simulink model "OML58_Cores"  (R2021b)
settings: Solver=ode4  StartTime=0.0  StopTime=inf  FixedStep=Ts  RelTol=1e-3  EnableMultiTasking=on
PostLoadFcn:
  | Ts = 50e-6;
InitFcn:
  | Ts = 50e-6;
undefined symbols (not defined in the file): I, Left, Right, type, V
libraries: spsSeriesRLCBranchLib x24, spsThreePhaseSeriesRLCLoadLib x12, spsThreePhaseSeriesRLCBranchLib x12, spsThreePhaseBreakerLib x12, artemis x10, spsGroundLib x8, rtlab x6, LafaeLib x6, spsThreePhaseTransformerTwoWindingsLib x5, spsThreePhaseVIMeasurementLib x5, spsPower3phInstantaneousLib x3, spsThreePhaseSourceLib x1
(part 1 of 3)
Description:
  | Model of a simple control system for use iin training.
settings Model: ARTEMISmethode_block_infos=$$__separator__$$OML58_Cores/ARTEMIS Guide$$__separator__$$  Creator=Paul Baracos  LastModifiedBy=lafae
settings SolverCC: AlgebraicLoopSolver=TrustRegion
settings DataIOCC: LimitDataPoints=on  SaveFormat=Array  SignalLoggingSaveFormat=ModelDataLogs  SaveOutput=off  SaveTime=off  ReturnWorkspaceOutputs=off  SignalLoggingName=sigsOut
settings OptimizationCC: BlockReduction=off  BooleanDataType=off  OptimizeBlockIOStorage=off  BufferReuse=off  ExpressionFolding=off  LocalBlockOutputs=off  InitFltsAndDblsToZero=on  LifeSpan=inf
settings DebuggingCC: SaveWithParameterizedLinksMsg=none  UnderspecifiedInitializationDetection=Classic  MergeDetectMultiDrivingBlocksExec=none  SignalResolutionControl=TryResolveAllWithWarning  MultiTaskDSMMsg=warning  MultiTaskCondExecSysMsg=none  FcnCallInpInsideContextMsg=warning  SFUnexpectedBacktrackingDiag=warning  SFNoUnconditionalDefaultTransitionDiag=warning  SFExecutionAtInitializationDiag=none  SFMachineParentedDataDiag=warning  ArithmeticOperatorsInVariantConditions=warning
settings HardwareCC: ProdBitPerPointer=32  ProdBitPerSizeT=32  ProdBitPerPtrDiffT=32  ProdLargestAtomicFloat=None  ProdIntDivRoundTo=Undefined  ProdEndianess=Unspecified  ProdWordSize=32  ProdHWDeviceType=32-bit Generic  TargetUnknown=on
settings ModelReferenceCC: PropagateSignalLabelsOutOfModel=off
settings SFSimCC: SimUseLocalCustomCode=off  CustomCodeUndefinedFunction=UseInterfaceOnly
settings RTWCC: RTWUseLocalCustomCode=off
settings CodeAppCC: StateflowObjectComments=on
settings GRTTargetCC: TargetFcnLib=ansi_tfl_tmw.mat  TargetLangStandard=C89/C90 (ANSI)  CombineOutputUpdateFcns=off  GRTInterface=on
settings ConfigComp: CovMetricSettings=dw  CovSaveCumulativeToWorkspaceVar=on  CovSaveSingleToWorkspaceVar=on  CovExternalEMLEnable=off

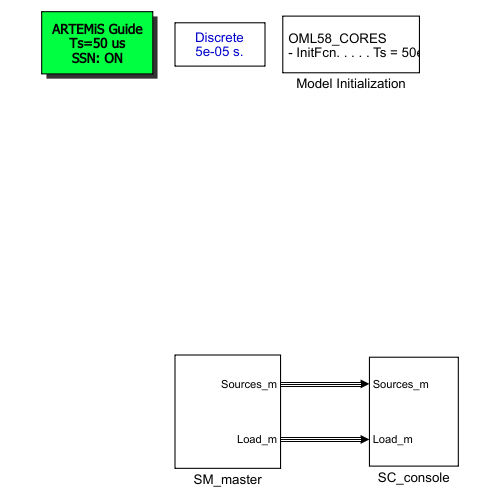
[thumbnail: Simulink's stored preview of the top-level diagram]
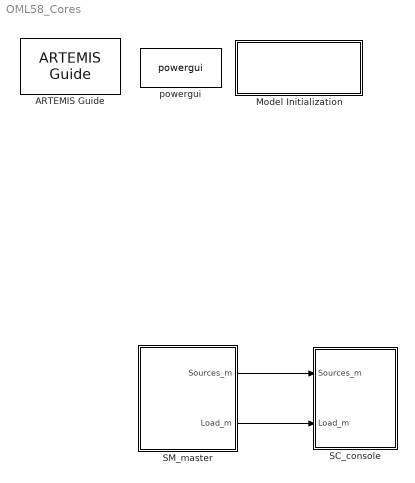
== system OML58_Cores ==
  ARTEMIS Guide : artemis/ARTEMIS/ARTEMIS Guide  Tag=art7.5  Description=New ARTEMiS block v 7.5b (R2015b+)  lock=on  Ts=Ts  ssn=on  opt=art5  dyna=off  nb_perm=4  RT_fullcomp=off  ssn_itvc=off  ssn_ivic=off  ssn_ext=off  ssn_solver=Art5 with Backward Euler nodal interface  iter_type=iSWITCH and iMOV only (default)  ssn_ImpulseLoopBlockedStateUpdate=5  ssn_mov_iter_number=5  ssn_switch_iter_number=3  ssn_lu_or_ldlt=LU (more robust)  ssn_nib_type_verify=off  ssn_use_lu=on  ssn_use_ldlt=off  ssn_impulse=on  ssn_quasimpulse=off  ssn_impulse_loop=5  paraExtinctionThy=off  Thy_Impulse=on  dtc=Off  dtc_opt=normal  ao=off  simtype=off  ct_mac=off  lin_mov=off  lsp=[0.001 2]  spike_skip=Disabled  dtc_extra=1  dtc_sws=normal  dtc_pied=0.5  SPSRulesBlock=SPSRules  tre=on  ctmm=off  LF=off  dpl_type=ARTEMiS DPL  rlc_type=off  custom_type=off  para=on  ssn_full_iteration=off  ssn_init_cond=block only
  Model Initialization : Subsystem  AncestorBlock=artemis/Tools /Misc/Model Initialization  mask(Model Functions){InitFcnX=Ts = 50e-6;, prel=off, posl=on, inif=on, strf=off}
      mask prompts: InitFcnX "Initialisation"; prel "Preload Function"; posl "PostLoad Function"; inif "InitFcn"; strf "StartFcn"
      mask init:
      | currentBlock = gcb;
      | root = bdroot(currentBlock);
      | 
      | if ~strcmp(get_param(root,'BlockDiagramType'),'library')
      |     if prel==1
      |         set_param(root, 'PreLoadFcn', InitFcnX);
      |     else
      |         set_param(root, 'PreLoadFcn', '');
      |     end
      |     if inif==1
      |         set_param(root, 'InitFcn', InitFcnX);
      |     else
      |         set_param(root, 'InitFcn', '');
      |     end
      |     if strf==1
      |         set_param(root, 'StartFcn', InitFcnX);
      |     else
      |         set_param(root, 'StartFcn', '');
      |     end
      |     if posl==1
      |         set_param(root, 'PostLoadFcn', InitFcnX);
      |     else
      |         set_param(root, 'PostLoadFcn', '');
      |     end
      | end
      | 
      | pos = get_param(currentBlock, 'Position');
      | width = pos(3) - pos(1); height = pos(4) - pos(2);
      | txt = [ upper(root) '\n' '- InitFcn. . . . . '  get_param(root, 'InitFcn') ];
      settings: CopyFcn=set_param(gcb,'LinkStatus','inactive')
      mask Display: text(5, height*0.5, txt, 'horizontalAlignment', 'left', 'verticalAlignment', 'middle') ;
  SC_console : Subsystem
  SM_master : Subsystem
  powergui : spspowerguiLib/powergui  Priority=1  SimulationMode=Discrete  SampleTime=Ts  frequency=60  Iterations=50  frequencyindice=0  Pbase=100e6  ErrMax=1e-4  UnitsV=kV  UnitsW=MW  buscounter=0  FunctionMessages=off  echomessages=off  EnableUseOfTLC=off  CurrentSourceSwitches=off  DisableSnubberDevices=off  DisableRonSwitches=off  DisableVfSwitches=off  DisplayEquations=off  AutomaticDiscreteSolvers=off  SolverType=Tustin/Backward Euler (TBE)  Interpol=off  ExternalGateDelay=off  methode=off  Ts=100  x0status=blocks  SPID=on  SwTol=0  HookPort=off  NonlinearTolerance=1e-4  nMaxIteration=100  ContinueOnMaxIteration=off  RestoreLinks=warning  ResistiveCurrentMeasurement=off  Frange=[0:2:500]  Ylog=off  Xlog=on  ShowGrid=off  save=off  variable=ZData  structure=0  ZoomFFT=off  StartTime=0.0  cycles=1  DisplayStyle=1  fundamental=60  FreqAxis=off  MaxFrequency=1000  frequencyindicesteady=1  RmsSteady=1  display=off
  wires:
  SM_master/1(Sources_m) -> SC_console/1(Sources_m)
  SM_master/2(Load_m) -> SC_console/2(Load_m)

== system OML58_Cores/Model Initialization ==

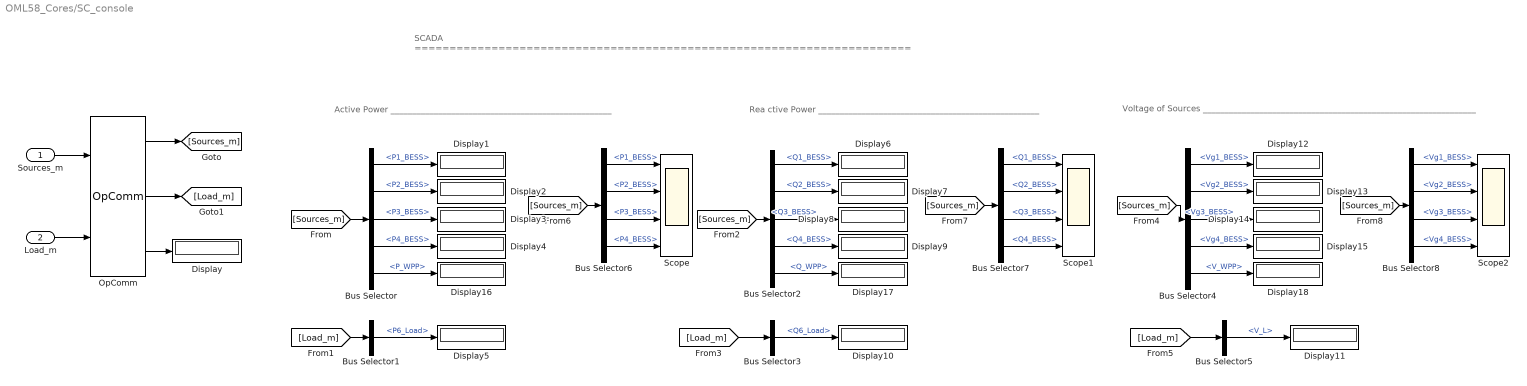
== system OML58_Cores/SC_console ==
  note: SCADA
      | =======================================================================
  note: Active Power
      | ___________________________________________________
  note: Rea ctive Power
      | ___________________________________________________
  note: Voltage of Sources
      | _______________________________________________________________
  Sources_m : Inport
  Load_m : Inport  Port=2
  Bus Selector : BusSelector  OutputSignals=BESS1.P1_BESS,BESS2.P2_BESS,BESS3.P3_BESS,BESS4.P4_BESS,WPP.P_WPP
  Bus Selector1 : BusSelector  OutputSignals=P6_Load
  Bus Selector2 : BusSelector  OutputSignals=BESS1.Q1_BESS,BESS2.Q2_BESS,BESS3.Q3_BESS,BESS4.Q4_BESS,WPP.Q_WPP
  Bus Selector3 : BusSelector  OutputSignals=Q6_Load
  Bus Selector4 : BusSelector  OutputSignals=BESS1.Vg1_BESS,BESS2.Vg2_BESS,BESS3.Vg3_BESS,BESS4.Vg4_BESS,WPP.V_WPP
  Bus Selector5 : BusSelector  OutputSignals=V_L
  Bus Selector6 : BusSelector  OutputSignals=BESS1.P1_BESS,BESS2.P2_BESS,BESS3.P3_BESS,BESS4.P4_BESS
  Bus Selector7 : BusSelector  OutputSignals=BESS1.Q1_BESS,BESS2.Q2_BESS,BESS3.Q3_BESS,BESS4.Q4_BESS
  Bus Selector8 : BusSelector  OutputSignals=BESS1.Vg1_BESS,BESS2.Vg2_BESS,BESS3.Vg3_BESS,BESS4.Vg4_BESS
  Display{,1..18} (19 alike) : Display
  OpComm : rtlab/OpComm  nbport=2  groupe_acq=1  subsys_rate=Ts  st=0  Synchronization=on  Interpolation=on  Threshold=1.0  Missed_Data=off  Sim_Time=on  Samples=off  dynSigOut=off  from_console=0  warning_done=off  writeOpCommFile=off  Offset=off
      settings: SourceProductName=RT-LAB
  Scope : Scope  NumInputPorts=4
  Scope1 : Scope  NumInputPorts=4
  Scope2 : Scope  NumInputPorts=4
  wires:
  Sources_m/1 -> OpComm/1
  Load_m/1 -> OpComm/2
  OpComm/1 -> [Sources_m]
  OpComm/2 -> [Load_m]
  OpComm/3 -> Display/1
  [Sources_m] -> Bus Selector/1
  Bus Selector/1 -> Display1/1  "<P1_BESS>"
  Bus Selector/2 -> Display2/1  "<P2_BESS>"
  Bus Selector/3 -> Display3/1  "<P3_BESS>"
  Bus Selector/4 -> Display4/1  "<P4_BESS>"
  [Load_m] -> Bus Selector1/1
  Bus Selector1/1 -> Display5/1  "<P6_Load>"
  Bus Selector3/1 -> Display10/1  "<Q6_Load>"
  [Load_m] -> Bus Selector3/1
  Bus Selector2/2 -> Display7/1  "<Q2_BESS>"
  Bus Selector2/1 -> Display6/1  "<Q1_BESS>"
  [Sources_m] -> Bus Selector2/1
  Bus Selector2/3 -> Display8/1  "<Q3_BESS>"
  Bus Selector2/4 -> Display9/1  "<Q4_BESS>"
  Bus Selector4/4 -> Display15/1  "<Vg4_BESS>"
  Bus Selector4/3 -> Display14/1  "<Vg3_BESS>"
  [Sources_m] -> Bus Selector4/1
  Bus Selector4/1 -> Display12/1  "<Vg1_BESS>"
  Bus Selector4/2 -> Display13/1  "<Vg2_BESS>"
  [Load_m] -> Bus Selector5/1
  Bus Selector5/1 -> Display11/1  "<V_L>"
  [Sources_m] -> Bus Selector6/1
  Bus Selector6/1 -> Scope/1  "<P1_BESS>"
  Bus Selector6/2 -> Scope/2  "<P2_BESS>"
  Bus Selector6/3 -> Scope/3  "<P3_BESS>"
  Bus Selector6/4 -> Scope/4  "<P4_BESS>"
  Bus Selector7/4 -> Scope1/4  "<Q4_BESS>"
  Bus Selector7/3 -> Scope1/3  "<Q3_BESS>"
  [Sources_m] -> Bus Selector7/1
  Bus Selector7/2 -> Scope1/2  "<Q2_BESS>"
  Bus Selector7/1 -> Scope1/1  "<Q1_BESS>"
  Bus Selector8/2 -> Scope2/2  "<Vg2_BESS>"
  [Sources_m] -> Bus Selector8/1
  Bus Selector8/3 -> Scope2/3  "<Vg3_BESS>"
  Bus Selector8/4 -> Scope2/4  "<Vg4_BESS>"
  Bus Selector8/1 -> Scope2/1  "<Vg1_BESS>"
  Bus Selector/5 -> Display16/1  "<P_WPP>"
  Bus Selector2/5 -> Display17/1  "<Q_WPP>"
  Bus Selector4/5 -> Display18/1  "<V_WPP>"
